simulink model "CONVEYOR"  (R2025a)
settings: Solver=VariableStepAuto  StartTime=0.0  StopTime=10.0  RelTol=1e-3
settings Model: Creator=adars  LastModifiedBy=adars

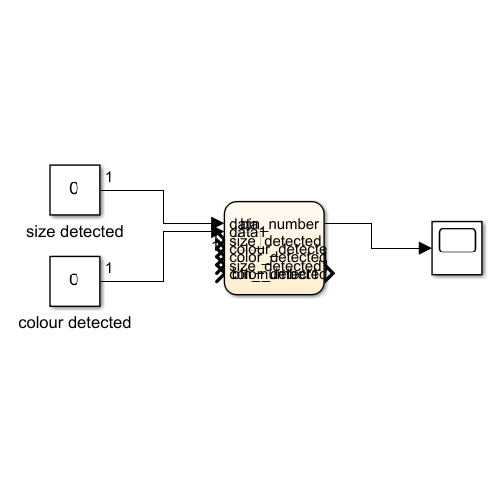
[thumbnail: Simulink's stored preview of the top-level diagram]
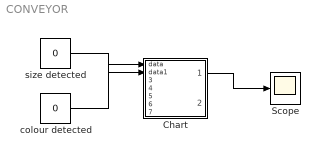
== system CONVEYOR ==
  Chart : Stateflow chart  TreatAsAtomicUnit=on
  Scope : Scope
  colour detected : Constant  Value=0
  size detected : Constant  Value=0
  wires:
  size detected/1 -> Chart/1(data)
  colour detected/1 -> Chart/2(data1)
  Chart/1(bin_number) -> Scope/1

== stateflow chart CONVEYOR/Chart ==
  state sorting
    if (size_detected == 0 && color_detected == 0)
    bin_number = 1;
    elseif (size_detected == 0 && color_detected == 1)
    bin_number = 2;
    elseif (size_detected == 1 && color_detected == 0)
    bin_number = 3;
    else
    bin_number = 4;
    end
  (default) -> sorting
  data: data input; data1 input; size_detected input; colour_detected input; bin_number output; color_detected input; size_detected1 input double; color_detected1 input double; bin_number1 output double
